simulink model "Assignment_01"  (R2023b)
settings: Solver=VariableStepAuto  StartTime=0.0  StopTime=17500  MaxStep=0.01  RelTol=1e-3
model workspace: external: MAT-File C:\Users\Frede\Documents\DTU\2024\Distributed Energy\Assignment 1\data_input_2024.mat (data not in the file)
undefined symbols (not defined in the file or in its folder): Ccell, Cth, NumCellsParallel, Rth, Tcell0
libraries: simulink x12
(part 1 of 2)
settings Model: Creator=matm  LastModifiedBy=Frede
settings SolverCC: ShapePreserveControl=EnableAll  AlgebraicLoopSolver=TrustRegion  SolverResetMethod=Robust
settings DataIOCC: ReturnWorkspaceOutputs=off
settings OptimizationCC: ReuseModelBlockBuffer=off
settings DebuggingCC: UnconnectedInputMsg=warning  UnconnectedOutputMsg=warning  UnconnectedLineMsg=warning  ArithmeticOperatorsInVariantConditions=warning
settings ModelReferenceCC: EnableRefExpFcnMdlSchedulingChecks=on
settings SFSimCC: SimUseLocalCustomCode=off  CustomCodeUndefinedFunction=UseInterfaceOnly
settings RTWCC: RTWUseLocalCustomCode=off  DLArmComputeVersion=19.05
settings CodeAppCC: StateflowObjectComments=on

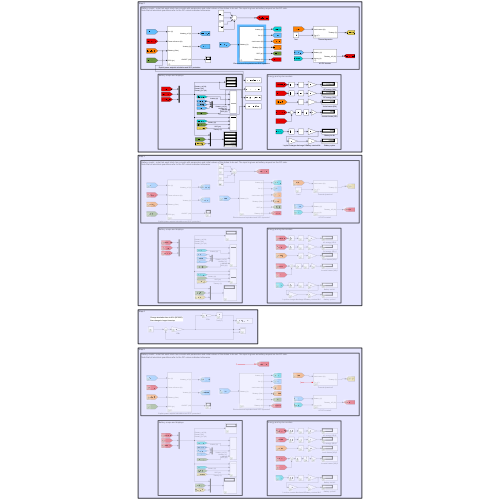
[thumbnail: Simulink's stored preview of the top-level diagram]
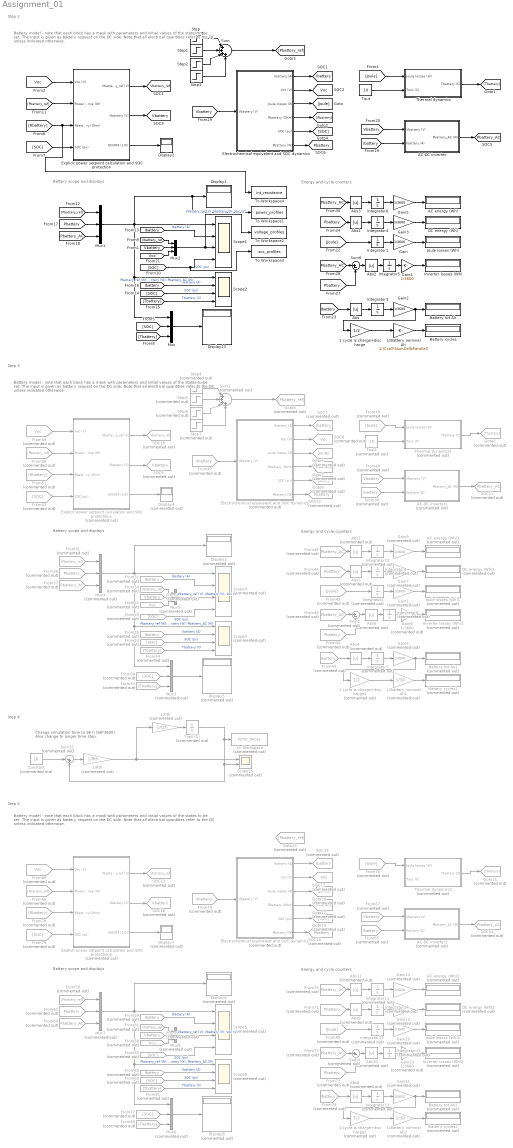
== system Assignment_01 ==
  note: Change simulation time to 96 h (96*3600).
      | Also change to longer time step.
  note: Step 2
  note: Battery model - note that each block has a mask with parameters and initial values of the states to be set. The input is given as battery request on the DC side.
      | Note that all electrical quantities refer to the DC unless indicated otherwise.
  note: Energy and cycle counters
  note: Battery scope and displays
  note: Step 4
  note: Battery scope and displays
  note: Battery model - note that each block has a mask with parameters and initial values of the states to be set. The input is given as battery request on the DC side.
      | Note that all electrical quantities refer to the DC unless indicated otherwise.
  note: Step 3
  note: Energy and cycle counters
  note: Battery model - note that each block has a mask with parameters and initial values of the states to be set. The input is given as battery request on the DC side.
      | Note that all electrical quantities refer to the DC unless indicated otherwise.
  note: Battery scope and displays
  note: Energy and cycle counters
  note: Step 5
  1 cycle is charge+discharge : Gain  Gain=1/2
  1 cycle is charge+discharge1 : Gain  Commented=on  Gain=1/2
  1 cycle is charge+discharge2 : Gain  Commented=on  Gain=1/2
  1/Battery nominal Ah : Gain  Gain=1/(Ccell*NumCellsParallel)
  1/Battery nominal Ah1 : Gain  Commented=on  Gain=1/30
  1/Battery nominal Ah2 : Gain  Commented=on  Gain=1/30
  1/Cth : Gain  Commented=on  Gain=-1/Cth
  1/Rth : Gain  Commented=on  Gain=1/Rth
  AC energy (Wh) : Display
  AC energy (Wh)1 : Display  Commented=on
  AC energy (Wh)2 : Display  Commented=on
  AC-DC inverter : Subsystem  mask{Inverter_Efficiency=0.95, Inverter_latency=0.1}
      mask prompts: Inverter_Efficiency "Inverter efficiency (pu)"; Inverter_latency "Inverter latency (s)"
  AC-DC inverter1 : Subsystem  Commented=on  mask{Inverter_Efficiency=0.95, Inverter_latency=0.1}
      mask prompts: Inverter_Efficiency "Inverter efficiency (pu)"; Inverter_latency "Inverter latency (s)"
  AC-DC inverter2 : Subsystem  Commented=on  mask{Inverter_Efficiency=0.95, Inverter_latency=0.1}
      mask prompts: Inverter_Efficiency "Inverter efficiency (pu)"; Inverter_latency "Inverter latency (s)"
  Abs{,1..3} (4 alike) : Abs  SaturateOnIntegerOverflow=off
  Abs{4..11} (8 alike) : Abs  Commented=on  SaturateOnIntegerOverflow=off
  Battery cycles : Display
  Battery cycles1 : Display  Commented=on
  Battery cycles2 : Display  Commented=on
  Battery tot Ah : Display
  Battery tot Ah1 : Display  Commented=on
  Battery tot Ah2 : Display  Commented=on
  Constant : Constant  Commented=on  Value=10
  DC energy (Wh) : Display
  DC energy (Wh)1 : Display  Commented=on
  DC energy (Wh)2 : Display  Commented=on
  Display1 : Display
  Display2 : Display
  Display23 : Display
  Display{3..8} (6 alike) : Display  Commented=on
  Electrochemical equivalent and SOC dynamics : Subsystem  mask{NumCellsSeries=96, NumCellsParallel=3, Ccell=58.8, SOC0=0.95}
      mask prompts: NumCellsSeries "Number of cells in Series"; NumCellsParallel "Number of cells in Parallel"; Ccell "Cell capacity (Ah)"; SOC0 "Initial state of charge (pu)"
  Electrochemical equivalent and SOC dynamics1 : Subsystem  Commented=on  mask{NumCellsSeries=96, NumCellsParallel=3, Ccell=58.8, SOC0=0.95}
      mask prompts: NumCellsSeries "Number of cells in Series"; NumCellsParallel "Number of cells in Parallel"; Ccell "Cell capacity (Ah)"; SOC0 "Initial state of charge (pu)"
  Electrochemical equivalent and SOC dynamics2 : Subsystem  Commented=on  mask{NumCellsSeries=96, NumCellsParallel=3, Ccell=58.8, SOC0=0.95}
      mask prompts: NumCellsSeries "Number of cells in Series"; NumCellsParallel "Number of cells in Parallel"; Ccell "Cell capacity (Ah)"; SOC0 "Initial state of charge (pu)"
  Explicit power setpoint calculation and SOC protection : Subsystem  mask{SOC_Max=0.95, SOC_Min=0.05, NumCellsSeries=96, CellVoltage_Max=4.2, CellVoltage_Min=2.9}
      mask prompts: SOC_Max "Max SOC (pu)"; SOC_Min "Min SOC (pu)"; NumCellsSeries "Number of cells in series"; CellVoltage_Max "Max cell voltage (V)"; CellVoltage_Min "Min cell voltage (V)"
      mask DialogControl DescTextVar Prompt: Power calculations and protections
  Explicit power setpoint calculation and SOC protection1 : Subsystem  Commented=on  mask{SOC_Max=0.95, SOC_Min=0.05, NumCellsSeries=96, CellVoltage_Max=4.2, CellVoltage_Min=2.9}
      mask prompts: SOC_Max "Max SOC (pu)"; SOC_Min "Min SOC (pu)"; NumCellsSeries "Number of cells in series"; CellVoltage_Max "Max cell voltage (V)"; CellVoltage_Min "Min cell voltage (V)"
      mask DialogControl DescTextVar Prompt: Power calculations and protections
  Explicit power setpoint calculation and SOC protection2 : Subsystem  Commented=on  mask{SOC_Max=0.95, SOC_Min=0.05, NumCellsSeries=96, CellVoltage_Max=4.2, CellVoltage_Min=2.9}
      mask prompts: SOC_Max "Max SOC (pu)"; SOC_Min "Min SOC (pu)"; NumCellsSeries "Number of cells in series"; CellVoltage_Max "Max cell voltage (V)"; CellVoltage_Min "Min cell voltage (V)"
      mask DialogControl DescTextVar Prompt: Power calculations and protections
  From{25,33,50,52,55,60,77,79} (8 alike) : From  Commented=on  GotoTag=SOC
  From{26,31,56,58} (4 alike) : From  Commented=on  GotoTag=Pbattery_ref
  From{3,40,47,57,67,74} (6 alike) : From  Commented=on  GotoTag=Vbattery  TagVisibility=global
  From{32,35,38,43,59,62,65,70} (8 alike) : From  Commented=on  GotoTag=Ibattery  TagVisibility=global
  From{34,53,61,80} (4 alike) : From  Commented=on  GotoTag=Tbattery
  From{36,44..45,63,71..72} (6 alike) : From  Commented=on  GotoTag=Pbattery  TagVisibility=global
  From{37,46,48,64,73,75} (6 alike) : From  Commented=on  GotoTag=Pbattery_AC  TagVisibility=global
  From{39,41,66,68} (4 alike) : From  Commented=on  GotoTag=Voc  TagVisibility=global
  From{42,49,69,76} (4 alike) : From  Commented=on  GotoTag=Joule
  From51 : From  Commented=on  GotoTag=Rbattery
  From54 : From  Commented=on  GotoTag=Vbattery_ref  TagVisibility=global
  From78 : From  Commented=on  GotoTag=Rbattery
  From81 : From  Commented=on  GotoTag=Vbattery_ref  TagVisibility=global
  Gain{,2..5} (5 alike) : Gain  Gain=1/3600
  Gain{1,6..14} (10 alike) : Gain  Commented=on  Gain=1/3600
  Goto10 : Goto  Commented=on  GotoTag=Joule
  Goto11 : Goto  Commented=on  GotoTag=Tbattery
  Goto12 : Goto  Commented=on  GotoTag=Rbattery
  Goto13 : Goto  Commented=on  GotoTag=Pbattery_ref
  Goto14 : Goto  Commented=on  GotoTag=SOC
  Goto5 : Goto  Commented=on  GotoTag=Joule
  Goto6 : Goto  Commented=on  GotoTag=Tbattery
  Goto7 : Goto  Commented=on  GotoTag=Rbattery
  Goto8 : Goto  Commented=on  GotoTag=Pbattery_ref
  Goto9 : Goto  Commented=on  GotoTag=SOC
  Integrator{1,3..6} (5 alike) : Integrator
  Integrator{2,7..15} (10 alike) : Integrator  Commented=on
  Inverter losses (Wh) : Display
  Inverter losses (Wh)1 : Display  Commented=on
  Inverter losses (Wh)2 : Display  Commented=on
  Joule losses (Wh) : Display
  Joule losses (Wh)1 : Display  Commented=on
  Joule losses (Wh)2 : Display  Commented=on
  Mux : Mux  Inputs=3
  Mux1 : Mux  Inputs=3
  Mux2 : Mux  Inputs=3
  Mux{3..8} (6 alike) : Mux  Commented=on  Inputs=3
  SOC10 : Goto  Commented=on  GotoTag=Vbattery_ref  TagVisibility=global
  SOC11 : Goto  Commented=on  GotoTag=Pbattery_AC  TagVisibility=global
  SOC12 : Goto  Commented=on  GotoTag=Pbattery  TagVisibility=global
  SOC13 : Goto  Commented=on  GotoTag=Vbattery_ref  TagVisibility=global
  SOC14 : Goto  Commented=on  GotoTag=Pbattery_AC  TagVisibility=global
  SOC15 : Goto  Commented=on  GotoTag=Pbattery  TagVisibility=global
  SOC16 : Goto  Commented=on  GotoTag=Ibattery  TagVisibility=global
  SOC17 : Goto  Commented=on  GotoTag=Voc  TagVisibility=global
  SOC18 : Goto  Commented=on  GotoTag=Vbattery  TagVisibility=global
  SOC7 : Goto  Commented=on  GotoTag=Ibattery  TagVisibility=global
  SOC8 : Goto  Commented=on  GotoTag=Voc  TagVisibility=global
  SOC9 : Goto  Commented=on  GotoTag=Vbattery  TagVisibility=global
  Scope1 : Scope  NumInputPorts=4
  Scope15 : Scope  Commented=on  NumInputPorts=2
  Scope2 : Scope  NumInputPorts=4
  Scope{3..6} (4 alike) : Scope  Commented=on  NumInputPorts=4
  Step : Step  Time=60  After=20000  SampleTime=0
  Step1 : Step  Time=10860  After=-20000  SampleTime=0
  Step2 : Step  Time=11000  After=-62000  SampleTime=0
  Step3 : Step  Time=14600  After=62000  SampleTime=0
  Step4 : Step  Commented=on  Time=60  After=20000  SampleTime=0
  Step5 : Step  Commented=on  Time=10860  After=-20000  SampleTime=0
  Step6 : Step  Commented=on  Time=11000  After=-62000  SampleTime=0
  Step7 : Step  Commented=on  Time=14600  After=62000  SampleTime=0
  Sum : Sum  Inputs=|++++
  Sum1 : Sum  Commented=on  Inputs=|++++
  Sum15 : Sum  Commented=on  Inputs=|-+
  Sum2 : Sum  Commented=on  Inputs=|+-
  Sum4 : Sum  Commented=on  Inputs=|+-
  Sum6 : Sum  Inputs=|+-
  Tcell (C) : Integrator  Commented=on  InitialCondition=40  ZeroCross=off
  Thermal dynamics : Subsystem  mask{Cth=309*1030, Rth=0.185}
      mask prompts: Cth "Thermal Capacitance (J/K)"; Rth "Thermal Resistance (K/W)"
      mask DialogControl DescTextVar Prompt: Thermal dynamic
  Thermal dynamics1 : Subsystem  Commented=on  mask{Cth=309*1030, Rth=0.185}
      mask prompts: Cth "Thermal Capacitance (J/K)"; Rth "Thermal Resistance (K/W)"
      mask DialogControl DescTextVar Prompt: Thermal dynamic
  Thermal dynamics2 : Subsystem  Commented=on  mask{Cth=309*1030, Rth=0.185}
      mask prompts: Cth "Thermal Capacitance (J/K)"; Rth "Thermal Resistance (K/W)"
      mask DialogControl DescTextVar Prompt: Thermal dynamic
  To Workspace : ToWorkspace  Commented=on  VariableName=temp_decay  SaveFormat=Timeseries  SampleTime=-1
  To Workspace1 : ToWorkspace  VariableName=power_profiles  SaveFormat=Timeseries  SampleTime=-1
  To Workspace2 : ToWorkspace  VariableName=voltage_profiles  SaveFormat=Timeseries  SampleTime=-1
  To Workspace3 : ToWorkspace  VariableName=soc_profiles  SaveFormat=Timeseries  SampleTime=-1
  To Workspace4 : ToWorkspace  VariableName=int_resistance  SaveFormat=Timeseries  SampleTime=-1
  Tout : Constant  Value=10
  Tout1 : Constant  Commented=on  Value=10
  tag scope: Ibattery=global, Pbattery=global, Pbattery_AC=global, Vbattery=global, Vbattery_ref=global, Voc=global
  wires:
  Integrator6/1 -> Gain5/1
  [Vbattery_ref] -> Mux2/1
  Step3/1 -> Sum/4
  [Voc] -> Mux2/3
  [Vbattery] -> AC-DC inverter/1(Vbattery (V))
  Gain4/1 -> Inverter losses (Wh)/1
  [Pbattery_AC] -> Mux1/3
  AC-DC inverter/1(Pbattery_AC (W)) -> [Pbattery_AC]
  Mux2/1 -> To Workspace2/1, Scope1/3  "Vbattery_ref (V); Vbattery (V); Voc (V)"
  Gain5/1 -> AC energy (Wh)/1
  Electrochemical equivalent and SOC dynamics/5(SOC (pu)) -> [SOC]
  [SOC] -> Scope2/3  "SOC (pu)"
  [Ibattery] -> Scope2/2  "Ibattery (A)"
  [Pbattery_AC] -> Sum6/1
  Integrator5/1 -> Gain4/1
  Abs3/1 -> Integrator6/1
  Step2/1 -> Sum/3
  Integrator4/1 -> Gain3/1
  Sum6/1 -> Abs2/1
  [Rbattery] -> To Workspace4/1, Explicit power setpoint calculation and SOC protection/3(Rbattery (Ohm))
  [Vbattery] -> Electrochemical equivalent and SOC dynamics/1(Vbattery (V))
  [Voc] -> Explicit power setpoint calculation and SOC protection/1(Voc (V))
  Gain2/1 -> 1 cycle is charge+discharge/1, Battery tot Ah/1
  Sum/1 -> [Pbattery_ref]
  [Joule] -> Thermal dynamics/1(Joule losses (W))
  Electrochemical equivalent and SOC dynamics/4(Rbattery (Ohm)) -> [Rbattery]
  [Pbattery_ref] -> Explicit power setpoint calculation and SOC protection/2(Power reference (W))
  Abs2/1 -> Integrator5/1
  Abs/1 -> Integrator3/1
  [SOC] -> To Workspace3/1, Scope1/4  "SOC (pu)"
  [Tbattery] -> Mux/3
  Thermal dynamics/1(Tbattery (C)) -> [Tbattery]
  [Pbattery_AC] -> Abs3/1
  [Joule] -> Integrator1/1
  [Tbattery] -> Scope2/4  "Tbattery (C)"
  [Pbattery] -> Mux1/2
  [Vbattery] -> Mux2/2
  Gain3/1 -> DC energy (Wh)/1
  [Pbattery_ref] -> Mux1/1
  Integrator1/1 -> Gain/1
  Tout/1 -> Thermal dynamics/2(Tout (C))
  Step1/1 -> Sum/2
  Gain/1 -> Joule losses (Wh)/1
  [Pbattery] -> Abs1/1
  Electrochemical equivalent and SOC dynamics/2(Voc (V)) -> [Voc]
  Step/1 -> Sum/1
  [Ibattery] -> Scope1/2  "Ibattery (A)"
  [SOC] -> Explicit power setpoint calculation and SOC protection/4(SOC (pu))
  Electrochemical equivalent and SOC dynamics/3(Joule losses (W)) -> [Joule]
  Electrochemical equivalent and SOC dynamics/6(Pbattery (W)) -> [Pbattery]
  Electrochemical equivalent and SOC dynamics/1(Ibattery (A)) -> [Ibattery]
  Explicit power setpoint calculation and SOC protection/1(Vbattery_ref (V)) -> [Vbattery_ref]
  Explicit power setpoint calculation and SOC protection/2(Vbattery (V)) -> [Vbattery]
  [Ibattery] -> Abs/1
  Integrator3/1 -> Gain2/1
  [Ibattery] -> AC-DC inverter/2(Ibattery (A))
  Abs1/1 -> Integrator4/1
  [SOC] -> Mux/2
  Explicit power setpoint calculation and SOC protection/3(ON/OFF (1/0)) -> Display2/1
  Mux/1 -> Display23/1
  Mux1/1 -> To Workspace1/1, Display1/1, Scope1/1, Scope2/1, Mux/1  "Pbattery_ref (W); Pbattery (W); Pbattery_AC (W)"
  [Pbattery] -> Sum6/2
  1/Battery nominal Ah/1 -> Battery cycles/1
  1 cycle is charge+discharge/1 -> 1/Battery nominal Ah/1
  Constant/1 -> Sum15/1
  1/Cth/1 -> Tcell (C)/1
  1/Rth/1 -> 1/Cth/1, Scope15/1
  Tcell (C)/1 -> To Workspace/1, Sum15/2, Scope15/2
  Sum15/1 -> 1/Rth/1
  1/Battery nominal Ah1/1 -> Battery cycles1/1
  From40/1 -> AC-DC inverter1/1(Vbattery (V))
  1 cycle is charge+discharge1/1 -> 1/Battery nominal Ah1/1
  Abs6/1 -> Integrator9/1
  From45/1 -> Sum2/2
  Electrochemical equivalent and SOC dynamics1/5(SOC (pu)) -> Goto9/1
  AC-DC inverter1/1(Pbattery_AC (W)) -> SOC11/1
  From33/1 -> Scope4/3  "SOC (pu)"
  Electrochemical equivalent and SOC dynamics1/4(Rbattery (Ohm)) -> Goto7/1
  From41/1 -> Mux5/3
  Abs5/1 -> Integrator8/1
  Integrator9/1 -> Gain8/1
  From42/1 -> Integrator2/1
  Abs4/1 -> Integrator7/1
  Mux5/1 -> Scope3/3  "Vbattery_ref (V); Vbattery (V); Voc (V)"
  Integrator7/1 -> Gain6/1
  Electrochemical equivalent and SOC dynamics1/1(Ibattery (A)) -> SOC7/1
  From50/1 -> Mux3/2
  Gain8/1 -> Inverter losses (Wh)1/1
  From39/1 -> Explicit power setpoint calculation and SOC protection1/1(Voc (V))
  From34/1 -> Scope4/4  "Tbattery (C)"
  Step4/1 -> Sum1/1
  Electrochemical equivalent and SOC dynamics1/2(Voc (V)) -> SOC8/1
  From37/1 -> Mux4/3
  From52/1 -> Explicit power setpoint calculation and SOC protection1/4(SOC (pu))
  From44/1 -> Abs5/1
  Gain1/1 -> Joule losses (Wh)1/1
  Step5/1 -> Sum1/2
  Tout1/1 -> Thermal dynamics1/2(Tout (C))
  From36/1 -> Mux4/2
  From32/1 -> Scope3/2  "Ibattery (A)"
  Integrator2/1 -> Gain1/1
  From31/1 -> Mux4/1
  Electrochemical equivalent and SOC dynamics1/3(Joule losses (W)) -> Goto5/1
  From3/1 -> Mux5/2
  Explicit power setpoint calculation and SOC protection1/1(Vbattery_ref (V)) -> SOC10/1
  Sum1/1 -> Goto8/1
  Abs7/1 -> Integrator10/1
  Gain9/1 -> AC energy (Wh)1/1
  From43/1 -> Abs4/1
  From54/1 -> Mux5/1
  From47/1 -> Electrochemical equivalent and SOC dynamics1/1(Vbattery (V))
  Electrochemical equivalent and SOC dynamics1/6(Pbattery (W)) -> SOC12/1
  Step7/1 -> Sum1/4
  Step6/1 -> Sum1/3
  From38/1 -> AC-DC inverter1/2(Ibattery (A))
  From53/1 -> Mux3/3
  Gain7/1 -> DC energy (Wh)1/1
  From26/1 -> Explicit power setpoint calculation and SOC protection1/2(Power reference (W))
  From35/1 -> Scope4/2  "Ibattery (A)"
  Integrator10/1 -> Gain9/1
  From46/1 -> Sum2/1
  Explicit power setpoint calculation and SOC protection1/2(Vbattery (V)) -> SOC9/1
  Gain6/1 -> 1 cycle is charge+discharge1/1, Battery tot Ah1/1
  Thermal dynamics1/1(Tbattery (C)) -> Goto6/1
  Explicit power setpoint calculation and SOC protection1/3(ON/OFF (1/0)) -> Display4/1
  Mux4/1 -> Display3/1, Scope3/1, Scope4/1, Mux3/1  "Pbattery_ref (W); Pbattery (W); Pbattery_AC (W)"
  From25/1 -> Scope3/4  "SOC (pu)"
  From48/1 -> Abs7/1
  Mux3/1 -> Display5/1
  From49/1 -> Thermal dynamics1/1(Joule losses (W))
  Integrator8/1 -> Gain7/1
  Sum2/1 -> Abs6/1
  From51/1 -> Explicit power setpoint calculation and SOC protection1/3(Rbattery (Ohm))
  From78/1 -> Explicit power setpoint calculation and SOC protection2/3(Rbattery (Ohm))
  Integrator14/1 -> Gain12/1
  From75/1 -> Abs11/1
  Sum4/1 -> Abs10/1
  From76/1 -> Thermal dynamics2/1(Joule losses (W))
  Mux6/1 -> Display8/1
  Mux7/1 -> Display6/1, Scope5/1, Scope6/1, Mux6/1  "Pbattery_ref (W); Pbattery (W); Pbattery_AC (W)"
  Explicit power setpoint calculation and SOC protection2/3(ON/OFF (1/0)) -> Display7/1
  Integrator13/1 -> Gain11/1
  Mux8/1 -> Scope5/3  "Vbattery_ref (V); Vbattery (V); Voc (V)"
  Electrochemical equivalent and SOC dynamics2/5(SOC (pu)) -> Goto14/1
  Electrochemical equivalent and SOC dynamics2/4(Rbattery (Ohm)) -> Goto12/1
  Abs10/1 -> Integrator15/1
  1/Battery nominal Ah2/1 -> Battery cycles2/1
  From72/1 -> Sum4/2
  Thermal dynamics2/1(Tbattery (C)) -> Goto11/1
  AC-DC inverter2/1(Pbattery_AC (W)) -> SOC14/1
  From65/1 -> AC-DC inverter2/2(Ibattery (A))
  Abs9/1 -> Integrator14/1
  Integrator11/1 -> Gain14/1
  Gain12/1 -> DC energy (Wh)2/1
  Explicit power setpoint calculation and SOC protection2/2(Vbattery (V)) -> SOC18/1
  From80/1 -> Mux6/3
  Electrochemical equivalent and SOC dynamics2/6(Pbattery (W)) -> SOC15/1
  1 cycle is charge+discharge2/1 -> 1/Battery nominal Ah2/1
  Explicit power setpoint calculation and SOC protection2/1(Vbattery_ref (V)) -> SOC13/1
  From73/1 -> Sum4/1
  From58/1 -> Mux7/1
  From62/1 -> Scope6/2  "Ibattery (A)"
  Abs8/1 -> Integrator13/1
  From70/1 -> Abs8/1
  ? -> Goto13/1
  From57/1 -> Mux8/2
  From56/1 -> Explicit power setpoint calculation and SOC protection2/2(Power reference (W))
  Abs11/1 -> Integrator11/1
  From68/1 -> Mux8/3
  Integrator12/1 -> Gain10/1
  From60/1 -> Scope6/3  "SOC (pu)"
  From81/1 -> Mux8/1
  From69/1 -> Integrator12/1
  From63/1 -> Mux7/2
  Gain10/1 -> Joule losses (Wh)2/1
  From59/1 -> Scope5/2  "Ibattery (A)"
  Gain11/1 -> 1 cycle is charge+discharge2/1, Battery tot Ah2/1
  Gain14/1 -> AC energy (Wh)2/1
  Electrochemical equivalent and SOC dynamics2/3(Joule losses (W)) -> Goto10/1
  From71/1 -> Abs9/1
  ? -> Thermal dynamics2/2(Tout (C))
  From66/1 -> Explicit power setpoint calculation and SOC protection2/1(Voc (V))
  From64/1 -> Mux7/3
  Electrochemical equivalent and SOC dynamics2/2(Voc (V)) -> SOC17/1
  From79/1 -> Explicit power setpoint calculation and SOC protection2/4(SOC (pu))
  Integrator15/1 -> Gain13/1
  From61/1 -> Scope6/4  "Tbattery (C)"
  From74/1 -> Electrochemical equivalent and SOC dynamics2/1(Vbattery (V))
  Gain13/1 -> Inverter losses (Wh)2/1
  From77/1 -> Mux6/2
  From55/1 -> Scope5/4  "SOC (pu)"
  Electrochemical equivalent and SOC dynamics2/1(Ibattery (A)) -> SOC16/1
  From67/1 -> AC-DC inverter2/1(Vbattery (V))

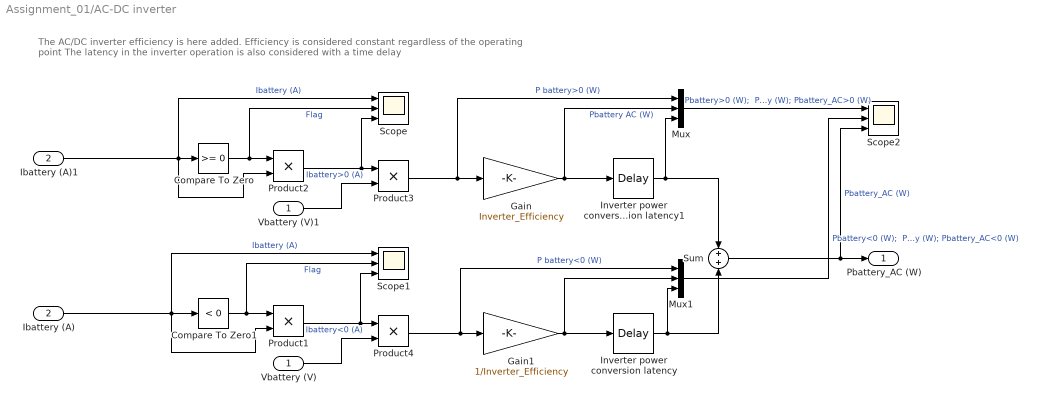
== system Assignment_01/AC-DC inverter ==
  note: The AC/DC inverter efficiency is here added. Efficiency is considered constant regardless of the operating point
      | The latency in the inverter operation is also considered with a time delay
  Vbattery (V) : Inport
  Ibattery (A) : Inport  Port=2
  Compare To Zero : simulink/Logic and Bit Operations/Compare To Zero  relop=>=  OutDataTypeStr=boolean
  Compare To Zero1 : simulink/Logic and Bit Operations/Compare To Zero  relop=<  OutDataTypeStr=boolean
  Gain : Gain  Gain=Inverter_Efficiency
  Gain1 : Gain  Gain=1/Inverter_Efficiency
  Ibattery (A)1 : InportShadow  Port=2
  Inverter power conversion latency : TransportDelay  DelayTime=Inverter_latency
  Inverter power conversion latency1 : TransportDelay  DelayTime=Inverter_latency
  Mux : Mux  Inputs=3
  Mux1 : Mux  Inputs=3
  Product{1..4} (4 alike) : Product
  Scope : Scope  NumInputPorts=3
  Scope1 : Scope  NumInputPorts=3
  Scope2 : Scope  NumInputPorts=3
  Sum : Sum
  Vbattery (V)1 : InportShadow
  Pbattery_AC (W) : Outport
  wires:
  Sum/1 -> Scope2/3, Pbattery_AC (W)/1  "Pbattery_AC (W)"
  Ibattery (A)1/1 -> Scope/1, Product2/2, Compare To Zero/1  "Ibattery (A)"
  Compare To Zero/1 -> Scope/2, Product2/1  "Flag"
  Product2/1 -> Product3/1, Scope/3  "Ibattery>0 (A)"
  Product3/1 -> Mux/1, Gain/1  "P battery>0 (W)"
  Vbattery (V)1/1 -> Product3/2
  Vbattery (V)/1 -> Product4/2
  Product1/1 -> Scope1/3, Product4/1  "Ibattery<0 (A)"
  Compare To Zero1/1 -> Scope1/2, Product1/1  "Flag"
  Ibattery (A)/1 -> Scope1/1, Product1/2, Compare To Zero1/1  "Ibattery (A)"
  Product4/1 -> Mux1/1, Gain1/1  "P battery<0 (W)"
  Gain/1 -> Mux/2, Inverter power conversion latency1/1  "Pbattery AC (W)"
  Gain1/1 -> Mux1/2, Inverter power conversion latency/1
  Inverter power conversion latency1/1 -> Mux/3, Sum/1
  Inverter power conversion latency/1 -> Mux1/3, Sum/2
  Mux/1 -> Scope2/1  "Pbattery>0 (W);  Pbattery_AC>0 no delay (W); Pbattery_AC>0 (W)"
  Mux1/1 -> Scope2/2  "Pbattery<0 (W);  Pbattery_AC<0 no delay (W); Pbattery_AC<0 (W)"

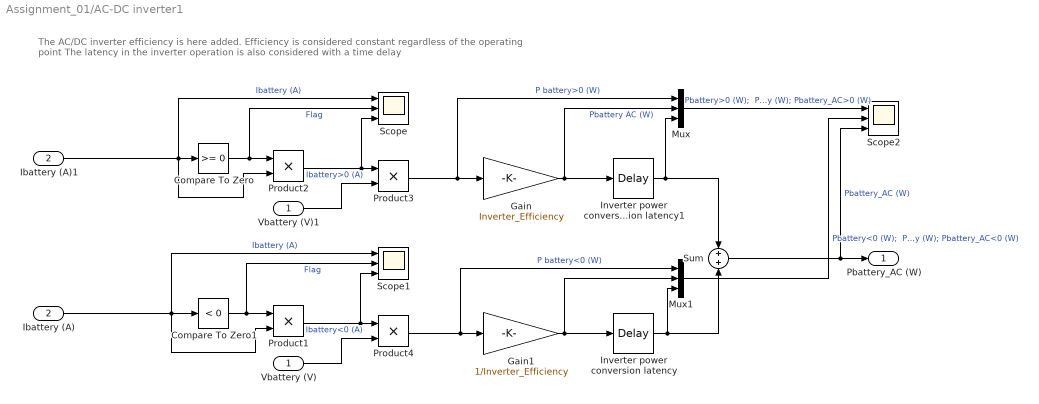
== system Assignment_01/AC-DC inverter1 ==
  note: The AC/DC inverter efficiency is here added. Efficiency is considered constant regardless of the operating point
      | The latency in the inverter operation is also considered with a time delay
  Vbattery (V) : Inport
  Ibattery (A) : Inport  Port=2
  Compare To Zero : simulink/Logic and Bit Operations/Compare To Zero  relop=>=  OutDataTypeStr=boolean
  Compare To Zero1 : simulink/Logic and Bit Operations/Compare To Zero  relop=<  OutDataTypeStr=boolean
  Gain : Gain  Gain=Inverter_Efficiency
  Gain1 : Gain  Gain=1/Inverter_Efficiency
  Ibattery (A)1 : InportShadow  Port=2
  Inverter power conversion latency : TransportDelay  DelayTime=Inverter_latency
  Inverter power conversion latency1 : TransportDelay  DelayTime=Inverter_latency
  Mux : Mux  Inputs=3
  Mux1 : Mux  Inputs=3
  Product{1..4} (4 alike) : Product
  Scope : Scope  NumInputPorts=3
  Scope1 : Scope  NumInputPorts=3
  Scope2 : Scope  NumInputPorts=3
  Sum : Sum
  Vbattery (V)1 : InportShadow
  Pbattery_AC (W) : Outport
  wires:
  Sum/1 -> Scope2/3, Pbattery_AC (W)/1  "Pbattery_AC (W)"
  Ibattery (A)1/1 -> Scope/1, Product2/2, Compare To Zero/1  "Ibattery (A)"
  Compare To Zero/1 -> Scope/2, Product2/1  "Flag"
  Product2/1 -> Product3/1, Scope/3  "Ibattery>0 (A)"
  Product3/1 -> Mux/1, Gain/1  "P battery>0 (W)"
  Vbattery (V)1/1 -> Product3/2
  Vbattery (V)/1 -> Product4/2
  Product1/1 -> Scope1/3, Product4/1  "Ibattery<0 (A)"
  Compare To Zero1/1 -> Scope1/2, Product1/1  "Flag"
  Ibattery (A)/1 -> Scope1/1, Product1/2, Compare To Zero1/1  "Ibattery (A)"
  Product4/1 -> Mux1/1, Gain1/1  "P battery<0 (W)"
  Gain/1 -> Mux/2, Inverter power conversion latency1/1  "Pbattery AC (W)"
  Gain1/1 -> Mux1/2, Inverter power conversion latency/1
  Inverter power conversion latency1/1 -> Mux/3, Sum/1
  Inverter power conversion latency/1 -> Mux1/3, Sum/2
  Mux/1 -> Scope2/1  "Pbattery>0 (W);  Pbattery_AC>0 no delay (W); Pbattery_AC>0 (W)"
  Mux1/1 -> Scope2/2  "Pbattery<0 (W);  Pbattery_AC<0 no delay (W); Pbattery_AC<0 (W)"

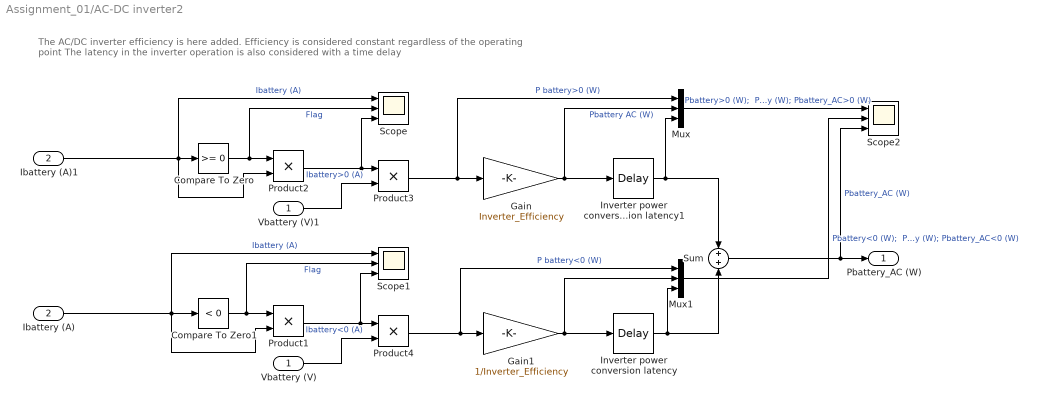
== system Assignment_01/AC-DC inverter2 ==
  note: The AC/DC inverter efficiency is here added. Efficiency is considered constant regardless of the operating point
      | The latency in the inverter operation is also considered with a time delay
  Vbattery (V) : Inport
  Ibattery (A) : Inport  Port=2
  Compare To Zero : simulink/Logic and Bit Operations/Compare To Zero  relop=>=  OutDataTypeStr=boolean
  Compare To Zero1 : simulink/Logic and Bit Operations/Compare To Zero  relop=<  OutDataTypeStr=boolean
  Gain : Gain  Gain=Inverter_Efficiency
  Gain1 : Gain  Gain=1/Inverter_Efficiency
  Ibattery (A)1 : InportShadow  Port=2
  Inverter power conversion latency : TransportDelay  DelayTime=Inverter_latency
  Inverter power conversion latency1 : TransportDelay  DelayTime=Inverter_latency
  Mux : Mux  Inputs=3
  Mux1 : Mux  Inputs=3
  Product{1..4} (4 alike) : Product
  Scope : Scope  NumInputPorts=3
  Scope1 : Scope  NumInputPorts=3
  Scope2 : Scope  NumInputPorts=3
  Sum : Sum
  Vbattery (V)1 : InportShadow
  Pbattery_AC (W) : Outport
  wires:
  Sum/1 -> Scope2/3, Pbattery_AC (W)/1  "Pbattery_AC (W)"
  Ibattery (A)1/1 -> Scope/1, Product2/2, Compare To Zero/1  "Ibattery (A)"
  Compare To Zero/1 -> Scope/2, Product2/1  "Flag"
  Product2/1 -> Product3/1, Scope/3  "Ibattery>0 (A)"
  Product3/1 -> Mux/1, Gain/1  "P battery>0 (W)"
  Vbattery (V)1/1 -> Product3/2
  Vbattery (V)/1 -> Product4/2
  Product1/1 -> Scope1/3, Product4/1  "Ibattery<0 (A)"
  Compare To Zero1/1 -> Scope1/2, Product1/1  "Flag"
  Ibattery (A)/1 -> Scope1/1, Product1/2, Compare To Zero1/1  "Ibattery (A)"
  Product4/1 -> Mux1/1, Gain1/1  "P battery<0 (W)"
  Gain/1 -> Mux/2, Inverter power conversion latency1/1  "Pbattery AC (W)"
  Gain1/1 -> Mux1/2, Inverter power conversion latency/1
  Inverter power conversion latency1/1 -> Mux/3, Sum/1
  Inverter power conversion latency/1 -> Mux1/3, Sum/2
  Mux/1 -> Scope2/1  "Pbattery>0 (W);  Pbattery_AC>0 no delay (W); Pbattery_AC>0 (W)"
  Mux1/1 -> Scope2/2  "Pbattery<0 (W);  Pbattery_AC<0 no delay (W); Pbattery_AC<0 (W)"

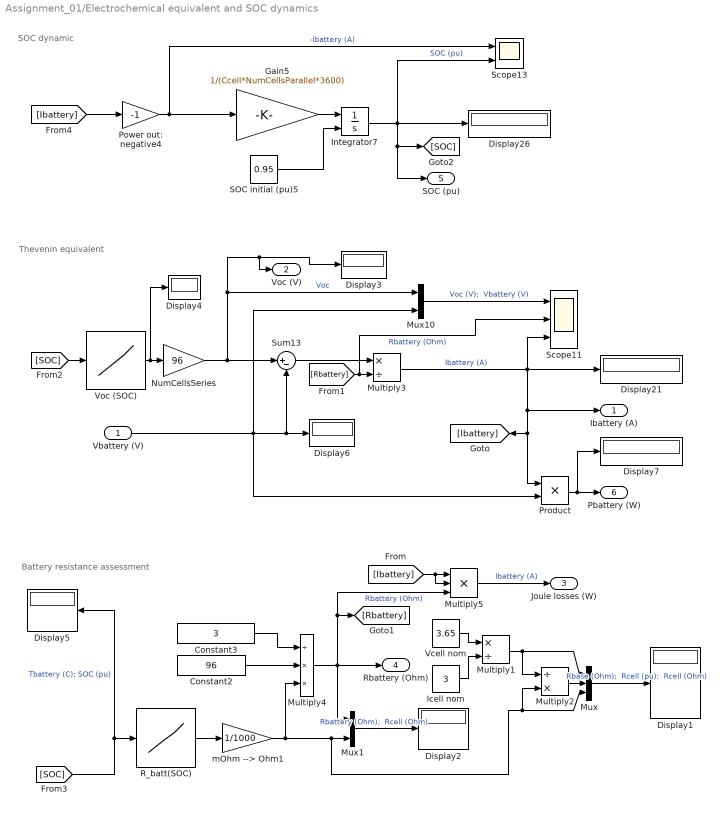
== system Assignment_01/Electrochemical equivalent and SOC dynamics ==
  note: SOC dynamic
  note: Battery resistance assessment
  note: Thevenin equivalent
  Vbattery (V) : Inport
  Constant2 : Constant  Value=96
  Constant3 : Constant  Value=3
  Display{1..7,21,26} (9 alike) : Display
  Gain5 : Gain  Gain=1/(Ccell*NumCellsParallel*3600)
  Icell nom : Constant  Value=3
  Integrator7 : Integrator  InitialConditionSource=external  InitialCondition=0.5  ZeroCross=off
  Multiply1 : Product  Inputs=*/
  Multiply2 : Product  Inputs=/*
  Multiply3 : Product  Inputs=*/
  Multiply4 : Product  Inputs=/**
  Multiply5 : Product  Inputs=***
  Mux : Mux  Inputs=3
  Mux1 : Mux  Inputs=2
  Mux10 : Mux  Inputs=2
  NumCellsSeries : Gain  Gain=96
  Power out: negative4 : Gain  Gain=-1
  Product : Product
  R_batt(SOC) : Lookup_n-D  NumberOfTableDimensions=1  BreakpointsForDimension1=[0.03 0.05 0.067 0.117 0.165 0.21 0.256 0.303 0.35 0.397 0.444 0.486 0.53 0.575 0.617 0.661 0.705 0.749 0.791 0.833 0.873 0.914 0.945 0.97]  Table=[4.14 4.14 4.14 4.28 3.84 3.72 3.71 3.82 4.05 4.43 4.83 4.78 4.72 3.84 3.59 3.71 3.99 4.33 4.66 4.97 5.32 5.32 5.32 5.32]  InternalRulePriority=Speed  RndMeth=Simplest
  SOC initial (pu)5 : Constant  Value=0.95
  Scope11 : Scope  NumInputPorts=3
  Scope13 : Scope  NumInputPorts=2
  Sum13 : Sum  Inputs=|+-
  Vcell nom : Constant  Value=3.65
  Voc (SOC) : Lookup_n-D  NumberOfTableDimensions=1  BreakpointsForDimension1=[0.03 0.05 0.067 0.117 0.165 0.21 0.256 0.303 0.35 0.397 0.444 0.486 0.53 0.575 0.617 0.661 0.705 0.749 0.791 0.833 0.873 0.914 0.945 0.97]  Table=[3.2 3.35 3.41 3.45 3.48 3.51 3.56 3.6 3.62 3.63 3.64 3.66 3.68 3.7 3.74 3.79 3.84 3.88 3.93 3.98 4.02 4.07 4.13 4.18]  InternalRulePriority=Speed  RndMeth=Simplest
  mOhm --> Ohm1 : Gain  Gain=1/1000
  Ibattery (A) : Outport  VectorParamsAs1DForOutWhenUnconnected=off
  Voc (V) : Outport  Port=2  VectorParamsAs1DForOutWhenUnconnected=off
  Joule losses (W) : Outport  Port=3  VectorParamsAs1DForOutWhenUnconnected=off
  Rbattery (Ohm) : Outport  Port=4  VectorParamsAs1DForOutWhenUnconnected=off
  SOC (pu) : Outport  Port=5  VectorParamsAs1DForOutWhenUnconnected=off
  Pbattery (W) : Outport  Port=6  VectorParamsAs1DForOutWhenUnconnected=off
  wires:
  Multiply3/1 -> Scope11/3, Display21/1, Product/1, [Ibattery], Ibattery (A)/1  "Ibattery (A)"
  [SOC] -> Voc (SOC)/1
  Mux10/1 -> Scope11/1  "Voc (V);  Vbattery (V)"
  Sum13/1 -> Multiply3/1
  Voc (SOC)/1 -> Display4/1, NumCellsSeries/1
  Vcell nom/1 -> Multiply1/1
  Icell nom/1 -> Multiply1/2
  R_batt(SOC)/1 -> mOhm --> Ohm1/1
  Multiply1/1 -> Mux/1, Multiply2/1
  Mux/1 -> Display1/1  "Rbase (Ohm);  Rcell (pu);  Rcell (Ohm)"
  Multiply2/1 -> Mux/2
  NumCellsSeries/1 -> Display3/1, Voc (V)/1, Mux10/1, Sum13/1  "Voc"
  Multiply5/1 -> Joule losses (W)/1  "Ibattery (A)"
  Mux1/1 -> Display2/1  "Rbattery (Ohm);  Rcell (Ohm)"
  Multiply4/1 -> Rbattery (Ohm)/1, [Rbattery], Multiply5/3, Mux1/1  "Rbattery (Ohm)"
  mOhm --> Ohm1/1 -> Mux/3, Multiply2/2, Mux1/2, Multiply4/3
  [SOC] -> Display5/1, R_batt(SOC)/1  "Tbattery (C); SOC (pu)"
  Constant3/1 -> Multiply4/1
  Constant2/1 -> Multiply4/2
  Vbattery (V)/1 -> Product/2, Mux10/2, Display6/1, Sum13/2
  SOC initial (pu)5/1 -> Integrator7/2
  Gain5/1 -> Integrator7/1
  [Ibattery] -> Power out: negative4/1
  Integrator7/1 -> SOC (pu)/1, [SOC], Scope13/2, Display26/1  "SOC (pu)"
  Power out: negative4/1 -> Gain5/1, Scope13/1  "-Ibattery (A)"
  [Ibattery] -> Multiply5/2, Multiply5/1
  [Rbattery] -> Scope11/2, Multiply3/2  "Rbattery (Ohm)"
  Product/1 -> Display7/1, Pbattery (W)/1

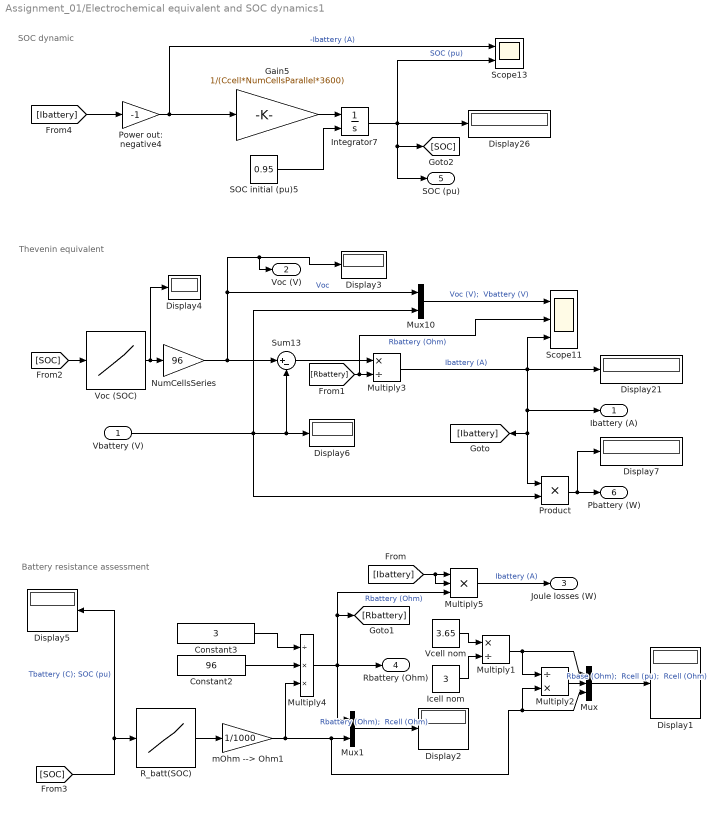
== system Assignment_01/Electrochemical equivalent and SOC dynamics1 ==
  note: SOC dynamic
  note: Battery resistance assessment
  note: Thevenin equivalent
  Vbattery (V) : Inport
  Constant2 : Constant  Value=96
  Constant3 : Constant  Value=3
  Display{1..7,21,26} (9 alike) : Display
  Gain5 : Gain  Gain=1/(Ccell*NumCellsParallel*3600)
  Icell nom : Constant  Value=3
  Integrator7 : Integrator  InitialConditionSource=external  InitialCondition=0.5  ZeroCross=off
  Multiply1 : Product  Inputs=*/
  Multiply2 : Product  Inputs=/*
  Multiply3 : Product  Inputs=*/
  Multiply4 : Product  Inputs=/**
  Multiply5 : Product  Inputs=***
  Mux : Mux  Inputs=3
  Mux1 : Mux  Inputs=2
  Mux10 : Mux  Inputs=2
  NumCellsSeries : Gain  Gain=96
  Power out: negative4 : Gain  Gain=-1
  Product : Product
  R_batt(SOC) : Lookup_n-D  NumberOfTableDimensions=1  BreakpointsForDimension1=[0.03 0.05 0.067 0.117 0.165 0.21 0.256 0.303 0.35 0.397 0.444 0.486 0.53 0.575 0.617 0.661 0.705 0.749 0.791 0.833 0.873 0.914 0.945 0.97]  Table=[4.14 4.14 4.14 4.28 3.84 3.72 3.71 3.82 4.05 4.43 4.83 4.78 4.72 3.84 3.59 3.71 3.99 4.33 4.66 4.97 5.32 5.32 5.32 5.32]  InternalRulePriority=Speed  RndMeth=Simplest
  SOC initial (pu)5 : Constant  Value=0.95
  Scope11 : Scope  NumInputPorts=3
  Scope13 : Scope  NumInputPorts=2
  Sum13 : Sum  Inputs=|+-
  Vcell nom : Constant  Value=3.65
  Voc (SOC) : Lookup_n-D  NumberOfTableDimensions=1  BreakpointsForDimension1=[0.03 0.05 0.067 0.117 0.165 0.21 0.256 0.303 0.35 0.397 0.444 0.486 0.53 0.575 0.617 0.661 0.705 0.749 0.791 0.833 0.873 0.914 0.945 0.97]  Table=[3.2 3.35 3.41 3.45 3.48 3.51 3.56 3.6 3.62 3.63 3.64 3.66 3.68 3.7 3.74 3.79 3.84 3.88 3.93 3.98 4.02 4.07 4.13 4.18]  InternalRulePriority=Speed  RndMeth=Simplest
  mOhm --> Ohm1 : Gain  Gain=1/1000
  Ibattery (A) : Outport  VectorParamsAs1DForOutWhenUnconnected=off
  Voc (V) : Outport  Port=2  VectorParamsAs1DForOutWhenUnconnected=off
  Joule losses (W) : Outport  Port=3  VectorParamsAs1DForOutWhenUnconnected=off
  Rbattery (Ohm) : Outport  Port=4  VectorParamsAs1DForOutWhenUnconnected=off
  SOC (pu) : Outport  Port=5  VectorParamsAs1DForOutWhenUnconnected=off
  Pbattery (W) : Outport  Port=6  VectorParamsAs1DForOutWhenUnconnected=off
  wires:
  Multiply3/1 -> Scope11/3, Display21/1, Product/1, [Ibattery], Ibattery (A)/1  "Ibattery (A)"
  [SOC] -> Voc (SOC)/1
  Mux10/1 -> Scope11/1  "Voc (V);  Vbattery (V)"
  Sum13/1 -> Multiply3/1
  Voc (SOC)/1 -> Display4/1, NumCellsSeries/1
  Vcell nom/1 -> Multiply1/1
  Icell nom/1 -> Multiply1/2
  R_batt(SOC)/1 -> mOhm --> Ohm1/1
  Multiply1/1 -> Mux/1, Multiply2/1
  Mux/1 -> Display1/1  "Rbase (Ohm);  Rcell (pu);  Rcell (Ohm)"
  Multiply2/1 -> Mux/2
  NumCellsSeries/1 -> Display3/1, Voc (V)/1, Mux10/1, Sum13/1  "Voc"
  Multiply5/1 -> Joule losses (W)/1  "Ibattery (A)"
  Mux1/1 -> Display2/1  "Rbattery (Ohm);  Rcell (Ohm)"
  Multiply4/1 -> Rbattery (Ohm)/1, [Rbattery], Multiply5/3, Mux1/1  "Rbattery (Ohm)"
  mOhm --> Ohm1/1 -> Mux/3, Multiply2/2, Mux1/2, Multiply4/3
  [SOC] -> Display5/1, R_batt(SOC)/1  "Tbattery (C); SOC (pu)"
  Constant3/1 -> Multiply4/1
  Constant2/1 -> Multiply4/2
  Vbattery (V)/1 -> Product/2, Mux10/2, Display6/1, Sum13/2
  SOC initial (pu)5/1 -> Integrator7/2
  Gain5/1 -> Integrator7/1
  [Ibattery] -> Power out: negative4/1
  Integrator7/1 -> SOC (pu)/1, [SOC], Scope13/2, Display26/1  "SOC (pu)"
  Power out: negative4/1 -> Gain5/1, Scope13/1  "-Ibattery (A)"
  [Ibattery] -> Multiply5/2, Multiply5/1
  [Rbattery] -> Scope11/2, Multiply3/2  "Rbattery (Ohm)"
  Product/1 -> Display7/1, Pbattery (W)/1

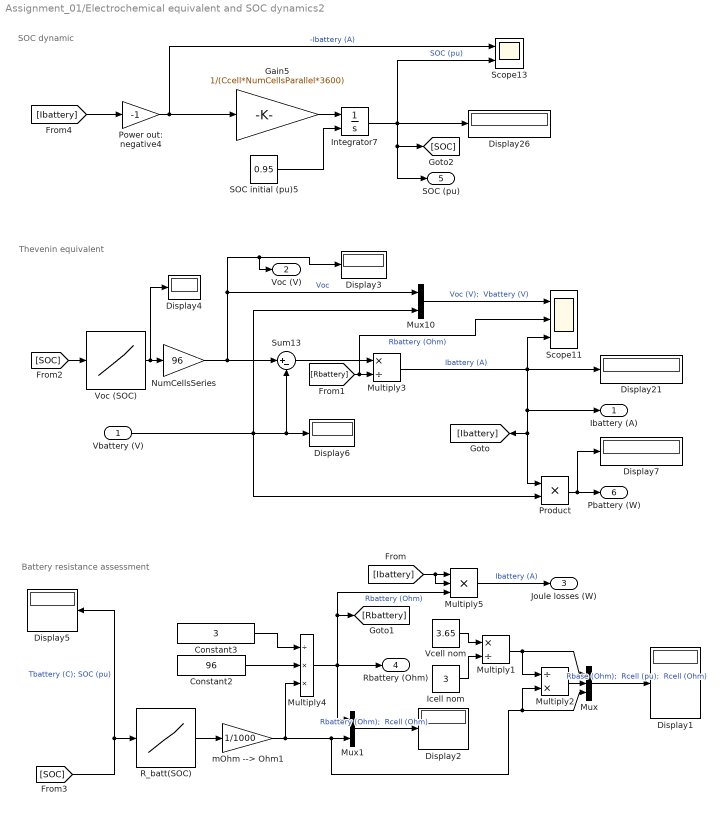
== system Assignment_01/Electrochemical equivalent and SOC dynamics2 ==
  note: SOC dynamic
  note: Battery resistance assessment
  note: Thevenin equivalent
  Vbattery (V) : Inport
  Constant2 : Constant  Value=96
  Constant3 : Constant  Value=3
  Display{1..7,21,26} (9 alike) : Display
  Gain5 : Gain  Gain=1/(Ccell*NumCellsParallel*3600)
  Icell nom : Constant  Value=3
  Integrator7 : Integrator  InitialConditionSource=external  InitialCondition=0.5  ZeroCross=off
  Multiply1 : Product  Inputs=*/
  Multiply2 : Product  Inputs=/*
  Multiply3 : Product  Inputs=*/
  Multiply4 : Product  Inputs=/**
  Multiply5 : Product  Inputs=***
  Mux : Mux  Inputs=3
  Mux1 : Mux  Inputs=2
  Mux10 : Mux  Inputs=2
  NumCellsSeries : Gain  Gain=96
  Power out: negative4 : Gain  Gain=-1
  Product : Product
  R_batt(SOC) : Lookup_n-D  NumberOfTableDimensions=1  BreakpointsForDimension1=[0.03 0.05 0.067 0.117 0.165 0.21 0.256 0.303 0.35 0.397 0.444 0.486 0.53 0.575 0.617 0.661 0.705 0.749 0.791 0.833 0.873 0.914 0.945 0.97]  Table=[4.14 4.14 4.14 4.28 3.84 3.72 3.71 3.82 4.05 4.43 4.83 4.78 4.72 3.84 3.59 3.71 3.99 4.33 4.66 4.97 5.32 5.32 5.32 5.32]  InternalRulePriority=Speed  RndMeth=Simplest
  SOC initial (pu)5 : Constant  Value=0.95
  Scope11 : Scope  NumInputPorts=3
  Scope13 : Scope  NumInputPorts=2
  Sum13 : Sum  Inputs=|+-
  Vcell nom : Constant  Value=3.65
  Voc (SOC) : Lookup_n-D  NumberOfTableDimensions=1  BreakpointsForDimension1=[0.03 0.05 0.067 0.117 0.165 0.21 0.256 0.303 0.35 0.397 0.444 0.486 0.53 0.575 0.617 0.661 0.705 0.749 0.791 0.833 0.873 0.914 0.945 0.97]  Table=[3.2 3.35 3.41 3.45 3.48 3.51 3.56 3.6 3.62 3.63 3.64 3.66 3.68 3.7 3.74 3.79 3.84 3.88 3.93 3.98 4.02 4.07 4.13 4.18]  InternalRulePriority=Speed  RndMeth=Simplest
  mOhm --> Ohm1 : Gain  Gain=1/1000
  Ibattery (A) : Outport  VectorParamsAs1DForOutWhenUnconnected=off
  Voc (V) : Outport  Port=2  VectorParamsAs1DForOutWhenUnconnected=off
  Joule losses (W) : Outport  Port=3  VectorParamsAs1DForOutWhenUnconnected=off
  Rbattery (Ohm) : Outport  Port=4  VectorParamsAs1DForOutWhenUnconnected=off
  SOC (pu) : Outport  Port=5  VectorParamsAs1DForOutWhenUnconnected=off
  Pbattery (W) : Outport  Port=6  VectorParamsAs1DForOutWhenUnconnected=off
  wires:
  Multiply3/1 -> Scope11/3, Display21/1, Product/1, [Ibattery], Ibattery (A)/1  "Ibattery (A)"
  [SOC] -> Voc (SOC)/1
  Mux10/1 -> Scope11/1  "Voc (V);  Vbattery (V)"
  Sum13/1 -> Multiply3/1
  Voc (SOC)/1 -> Display4/1, NumCellsSeries/1
  Vcell nom/1 -> Multiply1/1
  Icell nom/1 -> Multiply1/2
  R_batt(SOC)/1 -> mOhm --> Ohm1/1
  Multiply1/1 -> Mux/1, Multiply2/1
  Mux/1 -> Display1/1  "Rbase (Ohm);  Rcell (pu);  Rcell (Ohm)"
  Multiply2/1 -> Mux/2
  NumCellsSeries/1 -> Display3/1, Voc (V)/1, Mux10/1, Sum13/1  "Voc"
  Multiply5/1 -> Joule losses (W)/1  "Ibattery (A)"
  Mux1/1 -> Display2/1  "Rbattery (Ohm);  Rcell (Ohm)"
  Multiply4/1 -> Rbattery (Ohm)/1, [Rbattery], Multiply5/3, Mux1/1  "Rbattery (Ohm)"
  mOhm --> Ohm1/1 -> Mux/3, Multiply2/2, Mux1/2, Multiply4/3
  [SOC] -> Display5/1, R_batt(SOC)/1  "Tbattery (C); SOC (pu)"
  Constant3/1 -> Multiply4/1
  Constant2/1 -> Multiply4/2
  Vbattery (V)/1 -> Product/2, Mux10/2, Display6/1, Sum13/2
  SOC initial (pu)5/1 -> Integrator7/2
  Gain5/1 -> Integrator7/1
  [Ibattery] -> Power out: negative4/1
  Integrator7/1 -> SOC (pu)/1, [SOC], Scope13/2, Display26/1  "SOC (pu)"
  Power out: negative4/1 -> Gain5/1, Scope13/1  "-Ibattery (A)"
  [Ibattery] -> Multiply5/2, Multiply5/1
  [Rbattery] -> Scope11/2, Multiply3/2  "Rbattery (Ohm)"
  Product/1 -> Display7/1, Pbattery (W)/1

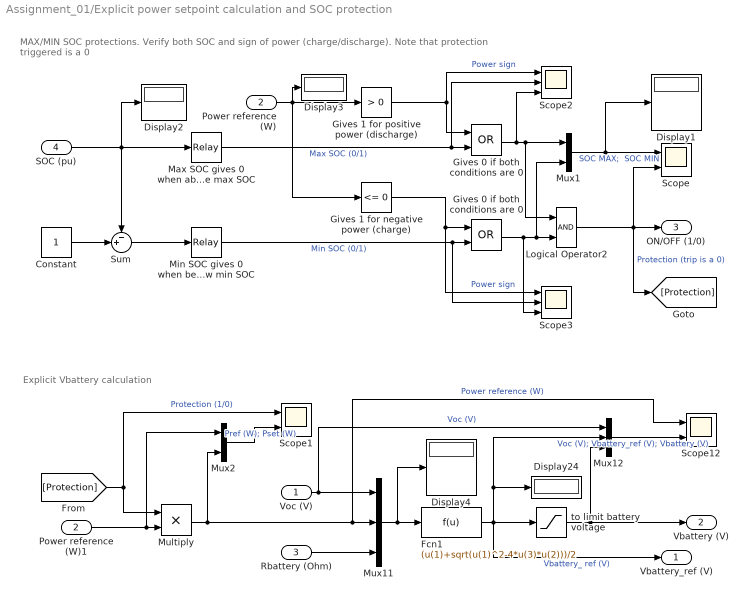
== system Assignment_01/Explicit power setpoint calculation and SOC protection ==
  note: Explicit Vbattery calculation
  note: MAX/MIN SOC protections. Verify both SOC and sign of power (charge/discharge). Note that protection triggered is a 0
  Voc (V) : Inport
  Power reference (W) : Inport  Port=2
  Rbattery (Ohm) : Inport  Port=3
  SOC (pu) : Inport  Port=4
  Constant : Constant
  Display{1..4,24} (5 alike) : Display
  Fcn1 : Fcn  Expr=(u(1)+sqrt(u(1)^2-4*u(3)*u(2)))/2
  "Gives 0 if both conditions are 0 " : Logic  Operator=OR  AllPortsSameDT=off  OutDataTypeStr=boolean
  "Gives 0 if both conditions are 0 " : Logic  Operator=OR  AllPortsSameDT=off  OutDataTypeStr=boolean
  Gives 1 for negative power (charge) : simulink/Logic and Bit Operations/Compare To Zero  relop=<=  OutDataTypeStr=boolean
  Gives 1 for positive power (discharge) : simulink/Logic and Bit Operations/Compare To Zero  relop=>  OutDataTypeStr=boolean
  Logical Operator2 : Logic  AllPortsSameDT=off  OutDataTypeStr=boolean
  "Max SOC gives 0 when above max SOC " : Relay  OnSwitchValue=SOC_Max  OffSwitchValue=SOC_Max-0.01  OnOutputValue=0  OffOutputValue=1
  Min SOC gives 0 when below min SOC : Relay  OnSwitchValue=1-SOC_Min  OffSwitchValue=1-(SOC_Min+0.01)  OnOutputValue=0  OffOutputValue=1
  Multiply : Product
  Mux1 : Mux  Inputs=2
  Mux11 : Mux  Inputs=3
  Mux12 : Mux  Inputs=3
  Mux2 : Mux  Inputs=2
  Power reference (W)1 : InportShadow  Port=2
  Scope : Scope  NumInputPorts=2
  Scope1 : Scope  NumInputPorts=2
  Scope12 : Scope  NumInputPorts=2
  Scope2 : Scope  NumInputPorts=3
  Scope3 : Scope  NumInputPorts=3
  Sum : Sum  Inputs=-+|
  to limit battery voltage : Saturate  UpperLimit=CellVoltage_Max*NumCellsSeries  LowerLimit=CellVoltage_Min*NumCellsSeries
  Vbattery_ref (V) : Outport  VectorParamsAs1DForOutWhenUnconnected=off
  Vbattery (V) : Outport  Port=2  VectorParamsAs1DForOutWhenUnconnected=off
  ON/OFF (1/0) : Outport  Port=3  VectorParamsAs1DForOutWhenUnconnected=off
  wires:
  Voc (V)/1 -> Mux12/1, Mux11/1  "Voc (V)"
  Fcn1/1 -> Vbattery_ref (V)/1, Mux12/2, Display24/1, to limit battery voltage/1  "Vbattery_ ref (V)"
  Mux11/1 -> Display4/1, Fcn1/1
  Mux12/1 -> Scope12/2  "Voc (V); Vbattery_ref (V); Vbattery (V)"
  Constant/1 -> Sum/2
  SOC (pu)/1 -> Display2/1, Sum/1, "Max SOC gives 0 when above max SOC "/1
  Sum/1 -> Min SOC gives 0 when below min SOC/1
  Gives 1 for negative power (charge)/1 -> "Gives 0 if both conditions are 0 "/1, Scope3/1  "Power sign"
  Gives 1 for positive power (discharge)/1 -> "Gives 0 if both conditions are 0 "/1, Scope2/1  "Power sign"
  Power reference (W)/1 -> Gives 1 for positive power (discharge)/1, Gives 1 for negative power (charge)/1, Display3/1
  "Gives 0 if both conditions are 0 "/1 -> Mux1/1, Logical Operator2/1, Scope2/3
  "Gives 0 if both conditions are 0 "/1 -> Mux1/2, Logical Operator2/2, Scope3/3
  Logical Operator2/1 -> [Protection], ON/OFF (1/0)/1, Scope/2  "Protection (trip is a 0)"
  Mux1/1 -> Display1/1, Scope/1  "SOC MAX;  SOC MIN"
  Power reference (W)1/1 -> Mux2/1, Multiply/2
  [Protection] -> Scope1/1, Multiply/1  "Protection (1/0)"
  Multiply/1 -> Mux2/2, Scope12/1, Mux11/2  "Power reference (W)"
  Rbattery (Ohm)/1 -> Mux11/3
  Mux2/1 -> Scope1/2  "Pref (W); Pset (W)"
  Min SOC gives 0 when below min SOC/1 -> Scope3/2, "Gives 0 if both conditions are 0 "/2  "Min SOC (0/1)"
  to limit battery voltage/1 -> Vbattery (V)/1, Mux12/3
  "Max SOC gives 0 when above max SOC "/1 -> Scope2/2, "Gives 0 if both conditions are 0 "/2  "Max SOC (0/1)"

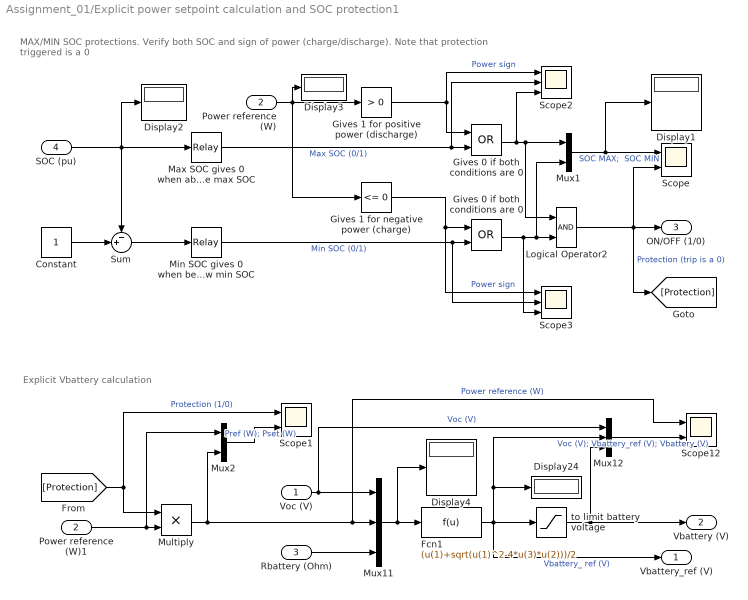
== system Assignment_01/Explicit power setpoint calculation and SOC protection1 ==
  note: Explicit Vbattery calculation
  note: MAX/MIN SOC protections. Verify both SOC and sign of power (charge/discharge). Note that protection triggered is a 0
  Voc (V) : Inport
  Power reference (W) : Inport  Port=2
  Rbattery (Ohm) : Inport  Port=3
  SOC (pu) : Inport  Port=4
  Constant : Constant
  Display{1..4,24} (5 alike) : Display
  Fcn1 : Fcn  Expr=(u(1)+sqrt(u(1)^2-4*u(3)*u(2)))/2
  "Gives 0 if both conditions are 0 " : Logic  Operator=OR  AllPortsSameDT=off  OutDataTypeStr=boolean
  "Gives 0 if both conditions are 0 " : Logic  Operator=OR  AllPortsSameDT=off  OutDataTypeStr=boolean
  Gives 1 for negative power (charge) : simulink/Logic and Bit Operations/Compare To Zero  relop=<=  OutDataTypeStr=boolean
  Gives 1 for positive power (discharge) : simulink/Logic and Bit Operations/Compare To Zero  relop=>  OutDataTypeStr=boolean
  Logical Operator2 : Logic  AllPortsSameDT=off  OutDataTypeStr=boolean
  "Max SOC gives 0 when above max SOC " : Relay  OnSwitchValue=SOC_Max  OffSwitchValue=SOC_Max-0.01  OnOutputValue=0  OffOutputValue=1
  Min SOC gives 0 when below min SOC : Relay  OnSwitchValue=1-SOC_Min  OffSwitchValue=1-(SOC_Min+0.01)  OnOutputValue=0  OffOutputValue=1
  Multiply : Product
  Mux1 : Mux  Inputs=2
  Mux11 : Mux  Inputs=3
  Mux12 : Mux  Inputs=3
  Mux2 : Mux  Inputs=2
  Power reference (W)1 : InportShadow  Port=2
  Scope : Scope  NumInputPorts=2
  Scope1 : Scope  NumInputPorts=2
  Scope12 : Scope  NumInputPorts=2
  Scope2 : Scope  NumInputPorts=3
  Scope3 : Scope  NumInputPorts=3
  Sum : Sum  Inputs=-+|
  to limit battery voltage : Saturate  UpperLimit=CellVoltage_Max*NumCellsSeries  LowerLimit=CellVoltage_Min*NumCellsSeries
  Vbattery_ref (V) : Outport  VectorParamsAs1DForOutWhenUnconnected=off
  Vbattery (V) : Outport  Port=2  VectorParamsAs1DForOutWhenUnconnected=off
  ON/OFF (1/0) : Outport  Port=3  VectorParamsAs1DForOutWhenUnconnected=off
  wires:
  Voc (V)/1 -> Mux12/1, Mux11/1  "Voc (V)"
  Fcn1/1 -> Vbattery_ref (V)/1, Mux12/2, Display24/1, to limit battery voltage/1  "Vbattery_ ref (V)"
  Mux11/1 -> Display4/1, Fcn1/1
  Mux12/1 -> Scope12/2  "Voc (V); Vbattery_ref (V); Vbattery (V)"
  Constant/1 -> Sum/2
  SOC (pu)/1 -> Display2/1, Sum/1, "Max SOC gives 0 when above max SOC "/1
  Sum/1 -> Min SOC gives 0 when below min SOC/1
  Gives 1 for negative power (charge)/1 -> "Gives 0 if both conditions are 0 "/1, Scope3/1  "Power sign"
  Gives 1 for positive power (discharge)/1 -> "Gives 0 if both conditions are 0 "/1, Scope2/1  "Power sign"
  Power reference (W)/1 -> Gives 1 for positive power (discharge)/1, Gives 1 for negative power (charge)/1, Display3/1
  "Gives 0 if both conditions are 0 "/1 -> Mux1/1, Logical Operator2/1, Scope2/3
  "Gives 0 if both conditions are 0 "/1 -> Mux1/2, Logical Operator2/2, Scope3/3
  Logical Operator2/1 -> [Protection], ON/OFF (1/0)/1, Scope/2  "Protection (trip is a 0)"
  Mux1/1 -> Display1/1, Scope/1  "SOC MAX;  SOC MIN"
  Power reference (W)1/1 -> Mux2/1, Multiply/2
  [Protection] -> Scope1/1, Multiply/1  "Protection (1/0)"
  Multiply/1 -> Mux2/2, Scope12/1, Mux11/2  "Power reference (W)"
  Rbattery (Ohm)/1 -> Mux11/3
  Mux2/1 -> Scope1/2  "Pref (W); Pset (W)"
  Min SOC gives 0 when below min SOC/1 -> Scope3/2, "Gives 0 if both conditions are 0 "/2  "Min SOC (0/1)"
  to limit battery voltage/1 -> Vbattery (V)/1, Mux12/3
  "Max SOC gives 0 when above max SOC "/1 -> Scope2/2, "Gives 0 if both conditions are 0 "/2  "Max SOC (0/1)"

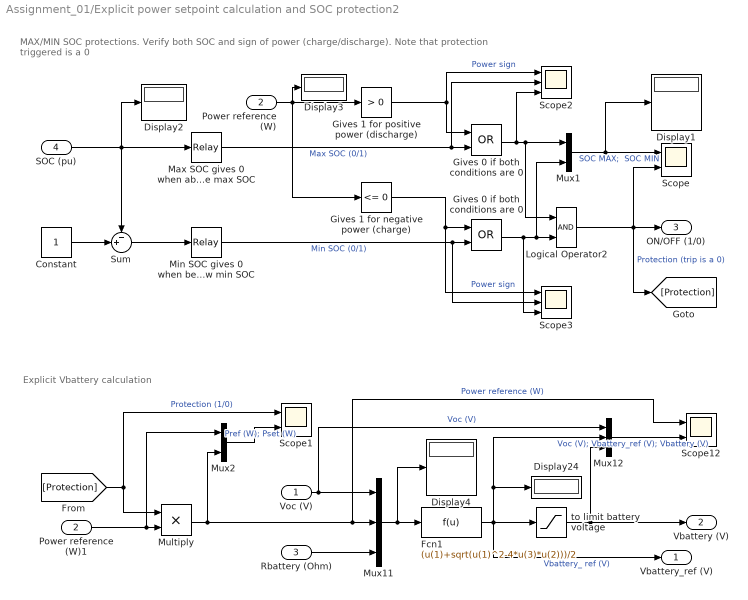
== system Assignment_01/Explicit power setpoint calculation and SOC protection2 ==
  note: Explicit Vbattery calculation
  note: MAX/MIN SOC protections. Verify both SOC and sign of power (charge/discharge). Note that protection triggered is a 0
  Voc (V) : Inport
  Power reference (W) : Inport  Port=2
  Rbattery (Ohm) : Inport  Port=3
  SOC (pu) : Inport  Port=4
  Constant : Constant
  Display{1..4,24} (5 alike) : Display
  Fcn1 : Fcn  Expr=(u(1)+sqrt(u(1)^2-4*u(3)*u(2)))/2
  "Gives 0 if both conditions are 0 " : Logic  Operator=OR  AllPortsSameDT=off  OutDataTypeStr=boolean
  "Gives 0 if both conditions are 0 " : Logic  Operator=OR  AllPortsSameDT=off  OutDataTypeStr=boolean
  Gives 1 for negative power (charge) : simulink/Logic and Bit Operations/Compare To Zero  relop=<=  OutDataTypeStr=boolean
  Gives 1 for positive power (discharge) : simulink/Logic and Bit Operations/Compare To Zero  relop=>  OutDataTypeStr=boolean
  Logical Operator2 : Logic  AllPortsSameDT=off  OutDataTypeStr=boolean
  "Max SOC gives 0 when above max SOC " : Relay  OnSwitchValue=SOC_Max  OffSwitchValue=SOC_Max-0.01  OnOutputValue=0  OffOutputValue=1
  Min SOC gives 0 when below min SOC : Relay  OnSwitchValue=1-SOC_Min  OffSwitchValue=1-(SOC_Min+0.01)  OnOutputValue=0  OffOutputValue=1
  Multiply : Product
  Mux1 : Mux  Inputs=2
  Mux11 : Mux  Inputs=3
  Mux12 : Mux  Inputs=3
  Mux2 : Mux  Inputs=2
  Power reference (W)1 : InportShadow  Port=2
  Scope : Scope  NumInputPorts=2
  Scope1 : Scope  NumInputPorts=2
  Scope12 : Scope  NumInputPorts=2
  Scope2 : Scope  NumInputPorts=3
  Scope3 : Scope  NumInputPorts=3
  Sum : Sum  Inputs=-+|
  to limit battery voltage : Saturate  UpperLimit=CellVoltage_Max*NumCellsSeries  LowerLimit=CellVoltage_Min*NumCellsSeries
  Vbattery_ref (V) : Outport  VectorParamsAs1DForOutWhenUnconnected=off
  Vbattery (V) : Outport  Port=2  VectorParamsAs1DForOutWhenUnconnected=off
  ON/OFF (1/0) : Outport  Port=3  VectorParamsAs1DForOutWhenUnconnected=off
  wires:
  Voc (V)/1 -> Mux12/1, Mux11/1  "Voc (V)"
  Fcn1/1 -> Vbattery_ref (V)/1, Mux12/2, Display24/1, to limit battery voltage/1  "Vbattery_ ref (V)"
  Mux11/1 -> Display4/1, Fcn1/1
  Mux12/1 -> Scope12/2  "Voc (V); Vbattery_ref (V); Vbattery (V)"
  Constant/1 -> Sum/2
  SOC (pu)/1 -> Display2/1, Sum/1, "Max SOC gives 0 when above max SOC "/1
  Sum/1 -> Min SOC gives 0 when below min SOC/1
  Gives 1 for negative power (charge)/1 -> "Gives 0 if both conditions are 0 "/1, Scope3/1  "Power sign"
  Gives 1 for positive power (discharge)/1 -> "Gives 0 if both conditions are 0 "/1, Scope2/1  "Power sign"
  Power reference (W)/1 -> Gives 1 for positive power (discharge)/1, Gives 1 for negative power (charge)/1, Display3/1
  "Gives 0 if both conditions are 0 "/1 -> Mux1/1, Logical Operator2/1, Scope2/3
  "Gives 0 if both conditions are 0 "/1 -> Mux1/2, Logical Operator2/2, Scope3/3
  Logical Operator2/1 -> [Protection], ON/OFF (1/0)/1, Scope/2  "Protection (trip is a 0)"
  Mux1/1 -> Display1/1, Scope/1  "SOC MAX;  SOC MIN"
  Power reference (W)1/1 -> Mux2/1, Multiply/2
  [Protection] -> Scope1/1, Multiply/1  "Protection (1/0)"
  Multiply/1 -> Mux2/2, Scope12/1, Mux11/2  "Power reference (W)"
  Rbattery (Ohm)/1 -> Mux11/3
  Mux2/1 -> Scope1/2  "Pref (W); Pset (W)"
  Min SOC gives 0 when below min SOC/1 -> Scope3/2, "Gives 0 if both conditions are 0 "/2  "Min SOC (0/1)"
  to limit battery voltage/1 -> Vbattery (V)/1, Mux12/3
  "Max SOC gives 0 when above max SOC "/1 -> Scope2/2, "Gives 0 if both conditions are 0 "/2  "Max SOC (0/1)"

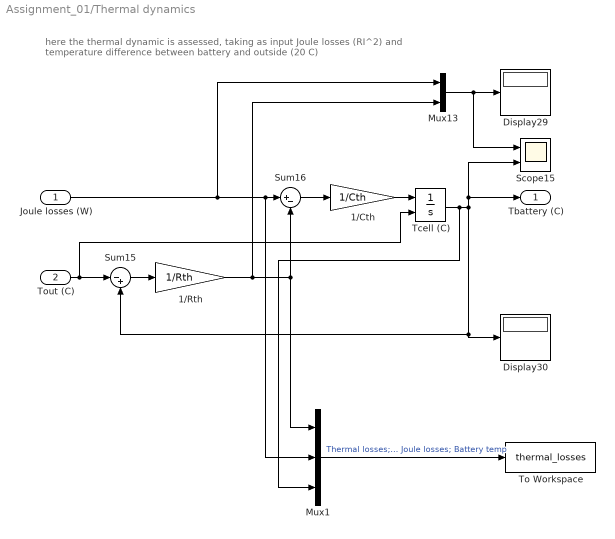
== system Assignment_01/Thermal dynamics ==
  note: here the thermal dynamic is assessed, taking as input Joule losses (RI^2)
      | and temperature difference between battery and outside (20 C)
  Joule losses (W) : Inport
  Tout (C) : Inport  Port=2
  1/Cth : Gain  Gain=1/Cth
  1/Rth : Gain  Gain=1/Rth
  Display29 : Display
  Display30 : Display
  Mux1 : Mux  Inputs=3
  Mux13 : Mux  Inputs=2
  Scope15 : Scope  NumInputPorts=2
  Sum15 : Sum  Inputs=|-+
  Sum16 : Sum  Inputs=|+-
  Tcell (C) : Integrator  InitialConditionSource=external  InitialCondition=Tcell0  ZeroCross=off
  To Workspace : ToWorkspace  VariableName=thermal_losses  SaveFormat=Timeseries  SampleTime=-1
  Tbattery (C) : Outport  VectorParamsAs1DForOutWhenUnconnected=off
  wires:
  1/Rth/1 -> Mux1/1, Sum16/2, Mux13/2
  Joule losses (W)/1 -> Mux13/1, Mux1/2, Sum16/1
  Sum16/1 -> 1/Cth/1
  Sum15/1 -> 1/Rth/1
  1/Cth/1 -> Tcell (C)/1
  Mux13/1 -> Display29/1, Scope15/1
  Tcell (C)/1 -> Mux1/3, Tbattery (C)/1, Scope15/2, Display30/1, Sum15/2
  Tout (C)/1 -> Tcell (C)/2, Sum15/1
  Mux1/1 -> To Workspace/1  "Thermal losses; Joule losses; Battery temp"

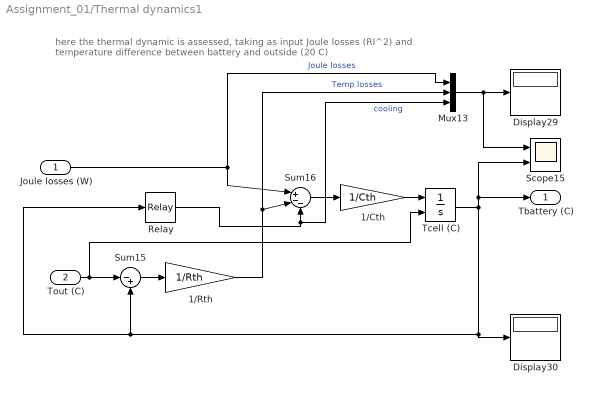
== system Assignment_01/Thermal dynamics1 ==
  note: here the thermal dynamic is assessed, taking as input Joule losses (RI^2)
      | and temperature difference between battery and outside (20 C)
  Joule losses (W) : Inport
  Tout (C) : Inport  Port=2
  1/Cth : Gain  Gain=1/Cth
  1/Rth : Gain  Gain=1/Rth
  Display29 : Display
  Display30 : Display
  Mux13 : Mux  Inputs=3
  Relay : Relay  OnSwitchValue=35  OffSwitchValue=25  OnOutputValue=4000
  Scope15 : Scope  NumInputPorts=2
  Sum15 : Sum  Inputs=|-+
  Sum16 : Sum  Inputs=|+--
  Tcell (C) : Integrator  InitialConditionSource=external  InitialCondition=Tcell0  ZeroCross=off
  Tbattery (C) : Outport  VectorParamsAs1DForOutWhenUnconnected=off
  wires:
  1/Rth/1 -> Sum16/2, Mux13/2  "Temp losses"
  Joule losses (W)/1 -> Sum16/1, Mux13/1  "Joule losses"
  Sum16/1 -> 1/Cth/1
  Sum15/1 -> 1/Rth/1
  1/Cth/1 -> Tcell (C)/1
  Mux13/1 -> Display29/1, Scope15/1
  Tcell (C)/1 -> Tbattery (C)/1, Scope15/2, Display30/1, Relay/1, Sum15/2
  Tout (C)/1 -> Tcell (C)/2, Sum15/1
  Relay/1 -> Mux13/3, Sum16/3  "cooling"
